simulink model "nonlinear"  (R2024a)
settings: Solver=VariableStepAuto  StartTime=0.0  StopTime=1  RelTol=1e-3
settings Model: Creator=perruquetti  LastModifiedBy=perruquetti

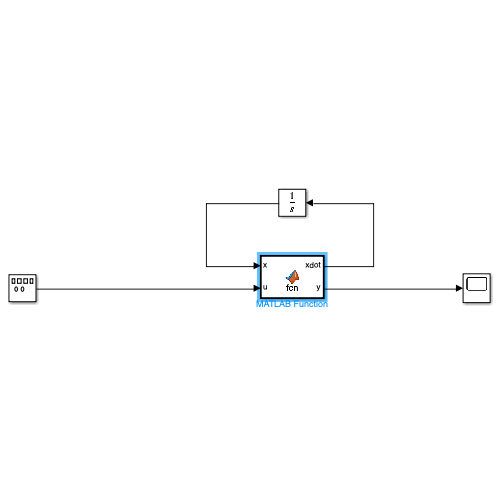
[thumbnail: Simulink's stored preview of the top-level diagram]
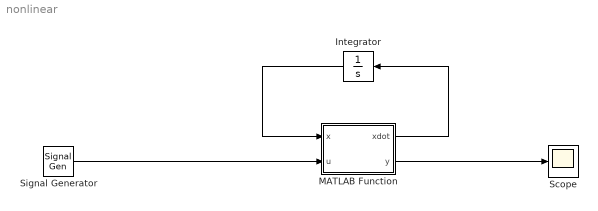
== system nonlinear ==
  Integrator : Integrator  InitialCondition="[0.012;  0; 0.84]"
  MATLAB Function : MATLAB Function  TreatAsAtomicUnit=on
  Scope : Scope
  Signal Generator : SignalGenerator  Amplitude=0.1  Units=rad/sec
  wires:
  MATLAB Function/1(xdot) -> Integrator/1
  Integrator/1 -> MATLAB Function/1(x)
  MATLAB Function/2(y) -> Scope/1
  Signal Generator/1 -> MATLAB Function/2(u)

== matlab function nonlinear/MATLAB Function ==
  data: x input; xdot output; u input; y output
function [xdot,y] = fcn(x,u)
% define your constants
    g = 9.81;
    m = 0.05;
    R = 1;
    L = 0.01;
    C = 0.0001; 
%   x1 = 0.012; %initial condition 1: displacement
%   x2 = 0;     %initial condition 2: velocity
%   x3 = 0.84;  %initial condition 3: acceleration

% nonlinear set of equations
    xdot = [x(2); g-((C/m)*(x(3)/x(1))^2); -((R/L) +(((2*C)/L)*(((x(2)*x(3))/((x(1))^2)))))] + [0;0;1/L]*u;

    y = x';
